simulink model "Hybrid_Skyhook_Groundhook_Control"  (R2020b)
settings: Solver=VariableStepAuto  StartTime=0.0  StopTime=10.0  RelTol=1e-3
values from neighbouring files (symbols this model uses):
  K = lqr( A, B(:,2), Q, R )    [Active_suspension_open_loop_setup.m]
  mu = 1    [Active_suspension_open_loop_setup.m]
settings Model: Creator=admin  LastModifiedBy=admin

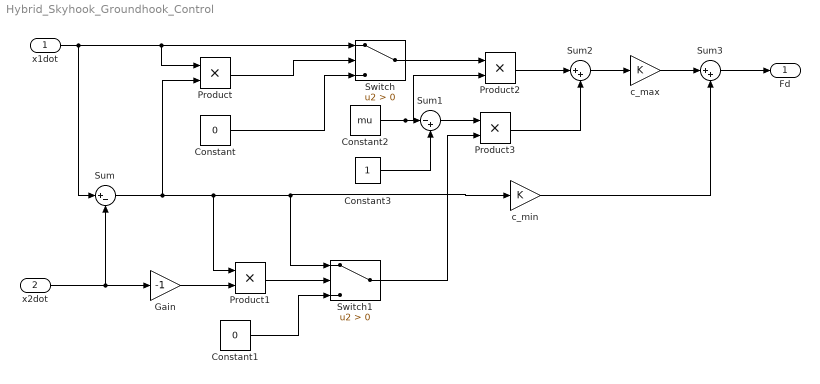
== system Hybrid_Skyhook_Groundhook_Control ==
  x1dot : Inport
  x2dot : Inport  Port=2
  Constant : Constant  Value=0
  Constant1 : Constant  Value=0
  Constant2 : Constant  Value=mu
  Constant3 : Constant
  Gain : Gain  Gain=-1
  Product{,1..3} (4 alike) : Product
  Sum : Sum  Inputs=|+-
  Sum1 : Sum  Inputs=|-+
  Sum2 : Sum  Inputs=|++
  Sum3 : Sum  Inputs=|++
  Switch : Switch  Criteria=u2 > Threshold
  Switch1 : Switch  Criteria=u2 > Threshold
  c_max : Gain  Gain=K
  c_min : Gain  Gain=K
  Fd : Outport
  wires:
  x1dot/1 -> Product/1, Switch/1, Sum/1
  x2dot/1 -> Sum/2, Gain/1
  Product/1 -> Switch/2
  Constant/1 -> Switch/3
  Gain/1 -> Product1/2
  Sum/1 -> c_min/1, Switch1/1, Product1/1, Product/2
  Product1/1 -> Switch1/2
  Constant1/1 -> Switch1/3
  Switch/1 -> Product2/1
  Constant2/1 -> Product2/2, Sum1/1
  Constant3/1 -> Sum1/2
  Sum1/1 -> Product3/1
  Switch1/1 -> Product3/2
  Product2/1 -> Sum2/1
  Product3/1 -> Sum2/2
  Sum2/1 -> c_max/1
  c_max/1 -> Sum3/1
  c_min/1 -> Sum3/2
  Sum3/1 -> Fd/1
